simulink library "ddm"  (R2021b)
settings: Solver=VariableStepAuto  StartTime=0.0  StopTime=10.0  RelTol=1e-3
undefined symbols (not defined in the file): ADDM_FrTMTqDev_X_Nm, ADDM_RrTMTqDev_X_Nm, ENUM_ADASACCSTA_ERROR, ENUM_ADASACCSTA_OFF, ENUM_ADASACCSTA_STANDBY, ENUM_ALLOWMOV_ALLOWREADY, ENUM_APS, ENUM_BRKSTA_ERROR, ENUM_BRKSTA_OFF, ENUM_BRKSTA_ON, ENUM_BRKSW_INVALID, ENUM_BRKSW_OFF, ENUM_BRKSW_ON, ENUM_CHGPREACTERRSTA_OBCPRE, ENUM_DCDCFAULTSTA_ANYFAULTLV1, ENUM_DCDCFAULTSTA_ANYFAULTLV2, ENUM_DRIVETRAIN_AWD, ENUM_DRIVETRAIN_FWD, ENUM_DRIVETRAIN_RWD, ENUM_EDUDRTSTA_NORMAL, ENUM_EPBERROR_FAILED, ENUM_EPBSTA_APPLIED, ENUM_EPBSTA_RELEASED, ENUM_ESCAPSSta_APSUNAVAILABLE, ENUM_GEARACTUALPOSN_INVALID, ENUM_GEARACTUALPOSN_P, ENUM_HVBATTREADYPRE_READY, ENUM_HWRESETSTA_HWRESETING, ENUM_MCUWARN_LV0, ENUM_MCUWARN_LV1, ENUM_MCUWARN_LV2, ENUM_MCUWARN_LV3, ENUM_MCUWARN_NOERROR, ENUM_OBCFAULTSTA_ANYFAULT, ENUM_PAS_R2F2, ENUM_PDFAULT_BATTPDFAIL, ENUM_PDFAULT_DCDCDISABLE, ENUM_PDFAULT_MCUDISABLE, ENUM_PDFAULT_MCUDISCHRG, ENUM_POWERSTA_OFF, ENUM_POWERSTA_ON, ENUM_POWERSTA_READY, ENUM_POWERSTA_STANDBY, ENUM_PRESSINDI_LOW, ENUM_PUFAULT_BATTUPFAIL, ENUM_PUFAULT_DCDCENABLEFAIL, ENUM_PUFAULT_PRECHRGCHKFAIL, ENUM_PUFAULT_SAFETYCHKFAIL, ENUM_PWRSTASW_OFF, ENUM_PWRSTASW_OFFA, ENUM_PWRSTASW_OFFCHVCHRG, ENUM_PWRSTASW_OFFCLVCHRG, ENUM_PWRSTASW_ON, ENUM_PWRSTASW_ONHVCHRG, ENUM_PWRSTASW_READY, ENUM_PWRSTASW_STANDBY, ENUM_RAPSErrWarnSta_NORMAL, ENUM_RAPSErrWarnSta_RAPSERRLV1, ENUM_SHIFTCOMMAND_P, ENUM_SHIFTERERRSTA_PBUTTONFAILURE ... (+471)
libraries: hcu_lib x540, simulink x3
(part 16 of 26)

== system ddm/DDM/DDM/VMC_DDM/Enabled Subsystem ==
  task_time_s : Inport
  VPMM_PowerSta_enum : Inport  Port=2
  VDDM_EPS1NoCom_flg : Inport  Port=3
  No_CAN1_BUS_OFF : Inport  Port=4
  DTC_clear_request : Inport  Port=5
  VTQD_GearActualPosn_enum : Inport  Port=6
  VDDM_EPSRCErr_flg : Inport  Port=7
  VDDM_EPSCSErr_flg : Inport  Port=8
  VINP_SASV_flg : Inport  Port=9
  EPS1 Checksum Error : Subsystem
  EPS1 Lost Comm : Subsystem
  "EPS1 Rolling Count Error " : Subsystem
  EPS1 Signal Error : Subsystem
  VDDM_EPS1NoComCFS_flg : Outport
  VDDM_EPS1NoComDTC_raw32 : Outport  Port=2
  VDDM_EPS1RCErrCFS_flg : Outport  Port=3
  VDDM_EPS1RCErrDTC_raw32 : Outport  Port=4
  VDDM_EPS1CSErrCFS_flg : Outport  Port=5
  VDDM_EPS1CSErrDTC_raw32 : Outport  Port=6
  VDDM_EPSSigErrCFS_flg : Outport  Port=7
  VDDM_EPSSigErrDTC_raw32 : Outport  Port=8
  wires:
  [task_time_s] -> EPS1 Lost Comm/1(task_time_s)
  [VPMM_PowerSta_enum] -> EPS1 Lost Comm/2(VPMM_PowerSta_enum)
  [VDDM_EPS1NoCom_flg] -> EPS1 Lost Comm/3(VDDM_EPS1NoCom_flg)
  [No_CAN1_BUS_OFF] -> EPS1 Lost Comm/4(No_CAN1_BUS_OFF)
  [DTC_clear_request] -> EPS1 Lost Comm/5(DTC_clear_request)
  [VTQD_GearActualPosn_enum] -> EPS1 Lost Comm/6(VTQD_GearActualPosn_enum)
  EPS1 Lost Comm/2(VDDM_EPS1NoComDTC_raw32) -> [VDDM_EPS1NoComDTC_raw32]
  EPS1 Lost Comm/1(VDDM_EPS1NoComCFS_flg) -> [VDDM_EPS1NoComCFS_flg]
  task_time_s/1 -> [task_time_s]
  VPMM_PowerSta_enum/1 -> [VPMM_PowerSta_enum]
  VDDM_EPS1NoCom_flg/1 -> [VDDM_EPS1NoCom_flg]
  No_CAN1_BUS_OFF/1 -> [No_CAN1_BUS_OFF]
  DTC_clear_request/1 -> [DTC_clear_request]
  VTQD_GearActualPosn_enum/1 -> [VTQD_GearActualPosn_enum]
  [VDDM_EPS1NoComCFS_flg] -> VDDM_EPS1NoComCFS_flg/1
  [VDDM_EPS1NoComDTC_raw32] -> VDDM_EPS1NoComDTC_raw32/1
  [task_time_s] -> "EPS1 Rolling Count Error "/1(task_time_s)
  [VDDM_EPSRCErr_flg] -> "EPS1 Rolling Count Error "/2(VDDM_EPSRCErr_flg)
  VDDM_EPSRCErr_flg/1 -> [VDDM_EPSRCErr_flg]
  [No_CAN1_BUS_OFF] -> "EPS1 Rolling Count Error "/3(No_CAN1_BUS_OFF)
  [VDDM_EPS1NoComCFS_flg] -> "EPS1 Rolling Count Error "/4(VDDM_EPS1NoComCFS_flg)
  [VPMM_PowerSta_enum] -> "EPS1 Rolling Count Error "/5(VPMM_PowerSta_enum)
  [DTC_clear_request] -> "EPS1 Rolling Count Error "/6(DTC_clear_request)
  [VTQD_GearActualPosn_enum] -> "EPS1 Rolling Count Error "/7(VTQD_GearActualPosn_enum)
  "EPS1 Rolling Count Error "/1(VDDM_EPS1RCErrCFS_flg) -> [VDDM_EPS1RCErrCFS_flg]
  "EPS1 Rolling Count Error "/2(VDDM_EPS1RCErrDTC_raw32) -> [VDDM_EPS1RCErrDTC_raw32]
  [VDDM_EPS1RCErrCFS_flg] -> VDDM_EPS1RCErrCFS_flg/1
  [VDDM_EPS1RCErrDTC_raw32] -> VDDM_EPS1RCErrDTC_raw32/1
  [task_time_s] -> EPS1 Checksum Error/1(task_time_s)
  [VDDM_EPSCSErr_flg] -> EPS1 Checksum Error/2(VDDM_EPSCSErr_flg)
  [No_CAN1_BUS_OFF] -> EPS1 Checksum Error/3(No_CAN1_BUS_OFF)
  [VDDM_EPS1NoComCFS_flg] -> EPS1 Checksum Error/4(VDDM_EPS1NoComCFS_flg)
  [VPMM_PowerSta_enum] -> EPS1 Checksum Error/5(VPMM_PowerSta_enum)
  [DTC_clear_request] -> EPS1 Checksum Error/6(DTC_clear_request)
  [VTQD_GearActualPosn_enum] -> EPS1 Checksum Error/7(VTQD_GearActualPosn_enum)
  VDDM_EPSCSErr_flg/1 -> [VDDM_EPSCSErr_flg]
  EPS1 Checksum Error/1(VDDM_EPS1CSErrCFS_flg) -> [VDDM_EPS1CSErrCFS_flg]
  EPS1 Checksum Error/2(VDDM_EPS1CSErrDTC_raw32) -> [VDDM_EPS1CSErrDTC_raw32]
  [VDDM_EPS1CSErrCFS_flg] -> VDDM_EPS1CSErrCFS_flg/1
  [VDDM_EPS1CSErrDTC_raw32] -> VDDM_EPS1CSErrDTC_raw32/1
  [task_time_s] -> EPS1 Signal Error/1(task_time_s)
  [VINP_SASV_flg] -> EPS1 Signal Error/2(VINP_SASV_flg)
  [No_CAN1_BUS_OFF] -> EPS1 Signal Error/3(No_CAN1_BUS_OFF)
  [VDDM_EPS1NoComCFS_flg] -> EPS1 Signal Error/4(VDDM_EPS1NoComCFS_flg)
  [VPMM_PowerSta_enum] -> EPS1 Signal Error/5(VPMM_PowerSta_enum)
  [DTC_clear_request] -> EPS1 Signal Error/6(DTC_clear_request)
  [VDDM_EPS1RCErrCFS_flg] -> EPS1 Signal Error/7(VDDM_EPS1RCErrCFS_flg)
  [VDDM_EPS1CSErrCFS_flg] -> EPS1 Signal Error/8(VDDM_EPS1CSErrCFS_flg)
  [VTQD_GearActualPosn_enum] -> EPS1 Signal Error/9(VTQD_GearActualPosn_enum)
  EPS1 Signal Error/1(VDDM_EPSSigErrCFS_flg) -> [VDDM_EPSSigErrCFS_flg]
  EPS1 Signal Error/2(VDDM_EPSSigErrDTC_raw32) -> [VDDM_EPSSigErrDTC_raw32]
  [VDDM_EPSSigErrCFS_flg] -> VDDM_EPSSigErrCFS_flg/1
  [VDDM_EPSSigErrDTC_raw32] -> VDDM_EPSSigErrDTC_raw32/1
  VINP_SASV_flg/1 -> [VINP_SASV_flg]

== system ddm/DDM/DDM/VMC_DDM/FCM1 ==
  task_time_s : Inport
  VDDM_FCM1NoCom_flg : Inport  Port=2
  VDDM_FCM1RCErr_flg : Inport  Port=3
  VDDM_FCM1CSErr_flg : Inport  Port=4
  No_CAN6_BUS_OFF : Inport  Port=5
  VPMM_PowerSta_enum : Inport  Port=6
  DTC_clear_request : Inport  Port=7
  "FCM1 Checksum Error " : Subsystem  AncestorBlock=ddm/DDM/DDM/VMC_DDM/FCM2/FCM2 Checksum Error
  FCM1 Lost Com : Subsystem  AncestorBlock=ddm/DDM/DDM/VMC_DDM/FCM2/FCM2 Lost Com
  "FCM1 Rolling Count Error " : Subsystem  AncestorBlock=ddm/DDM/DDM/VMC_DDM/FCM2/FCM2 Rolling Count Error
  VDDM_FCM1NoComCFS_flg : Outport
  VDDM_FCM1RCErrCFS_flg : Outport  Port=2
  VDDM_FCM1CSErrCFS_flg : Outport  Port=3
  VDDM_FCM1NoComDTC_raw32 : Outport  Port=4
  VDDM_FCM1RCErrDTC_raw32 : Outport  Port=5
  VDDM_FCM1CSErrDTC_raw32 : Outport  Port=6
  wires:
  [VDDM_FCM1CSErrDTC_raw32] -> VDDM_FCM1CSErrDTC_raw32/1
  [VDDM_FCM1RCErrDTC_raw32] -> VDDM_FCM1RCErrDTC_raw32/1
  [VDDM_FCM1NoComDTC_raw32] -> VDDM_FCM1NoComDTC_raw32/1
  "FCM1 Checksum Error "/2(VDDM_FCM1CSErrDTC_raw32) -> [VDDM_FCM1CSErrDTC_raw32]
  "FCM1 Rolling Count Error "/2(VDDM_FCM1RCErrDTC_raw32) -> [VDDM_FCM1RCErrDTC_raw32]
  FCM1 Lost Com/2(VDDM_FCM1NoComDTC_raw32) -> [VDDM_FCM1NoComDTC_raw32]
  "FCM1 Checksum Error "/1(VDDM_FCM1CSErrCFS_flg) -> [VDDM_FCM1CSErrCFS_flg]
  [VDDM_FCM1NoComCFS_flg] -> "FCM1 Checksum Error "/4(VDDM_FCM1NoComCFS_flg)
  [VDDM_FCM1CSErr_flg] -> "FCM1 Checksum Error "/2(VDDM_FCM1CSErr_flg)
  [No_CAN6_BUS_OFF] -> "FCM1 Checksum Error "/3(No_CAN6_BUS_OFF)
  [VPMM_PowerSta_enum] -> "FCM1 Checksum Error "/5(VPMM_PowerSta_enum)
  [DTC_clear_request] -> "FCM1 Checksum Error "/6(DTC_clear_request)
  [task_time_s] -> "FCM1 Checksum Error "/1(task_time_s)
  [task_time_s] -> "FCM1 Rolling Count Error "/1(task_time_s)
  task_time_s/1 -> [task_time_s]  "task_time_s"
  [task_time_s] -> FCM1 Lost Com/1(task_time_s)
  VDDM_FCM1CSErr_flg/1 -> [VDDM_FCM1CSErr_flg]
  VDDM_FCM1RCErr_flg/1 -> [VDDM_FCM1RCErr_flg]
  [VDDM_FCM1RCErrCFS_flg] -> VDDM_FCM1RCErrCFS_flg/1
  [VDDM_FCM1CSErrCFS_flg] -> VDDM_FCM1CSErrCFS_flg/1
  [VDDM_FCM1NoComCFS_flg] -> VDDM_FCM1NoComCFS_flg/1
  "FCM1 Rolling Count Error "/1(VDDM_FCM1RCErrCFS_flg) -> [VDDM_FCM1RCErrCFS_flg]
  [DTC_clear_request] -> "FCM1 Rolling Count Error "/6(DTC_clear_request)
  [VPMM_PowerSta_enum] -> "FCM1 Rolling Count Error "/5(VPMM_PowerSta_enum)
  [No_CAN6_BUS_OFF] -> "FCM1 Rolling Count Error "/3(No_CAN6_BUS_OFF)
  [VDDM_FCM1RCErr_flg] -> "FCM1 Rolling Count Error "/2(VDDM_FCM1RCErr_flg)
  [VDDM_FCM1NoComCFS_flg] -> "FCM1 Rolling Count Error "/4(VDDM_FCM1NoComCFS_flg)
  FCM1 Lost Com/1(VDDM_FCM1NoComCFS_flg) -> [VDDM_FCM1NoComCFS_flg]
  [DTC_clear_request] -> FCM1 Lost Com/5(DTC_clear_request)
  [VPMM_PowerSta_enum] -> FCM1 Lost Com/4(VPMM_PowerSta_enum)
  [No_CAN6_BUS_OFF] -> FCM1 Lost Com/3(No_CAN6_BUS_OFF)
  DTC_clear_request/1 -> [DTC_clear_request]
  VPMM_PowerSta_enum/1 -> [VPMM_PowerSta_enum]
  No_CAN6_BUS_OFF/1 -> [No_CAN6_BUS_OFF]
  [VDDM_FCM1NoCom_flg] -> FCM1 Lost Com/2(VDDM_FCM1NoCom_flg)
  VDDM_FCM1NoCom_flg/1 -> [VDDM_FCM1NoCom_flg]

== system ddm/DDM/DDM/VMC_DDM/FCMACC Signal Error ==
  task_time_s : Inport
  VDDM_FCM1NoComCFS_flg : Inport  Port=2
  VDDM_FCM1RCErrCFS_flg : Inport  Port=3
  VDDM_FCM1CSErrCFS_flg : Inport  Port=4
  No_CAN6_BUS_OFF : Inport  Port=5
  VPMM_PowerSta_enum : Inport  Port=6
  VINP_ADASACCSta_enum : Inport  Port=7
  DTC_clear_request : Inport  Port=8
  VTQD_ExternalTqAllow_flg : Inport  Port=9
  VTQD_ExtDoorAllow_flg : Inport  Port=10
  "FCMACC Signal Error " : Subsystem
  VDDM_FCMACCSigErrCFS_flg : Outport
  VDDM_FCMACCSigErrDetDTC_raw32 : Outport  Port=2
  wires:
  VDDM_FCM1CSErrCFS_flg/1 -> [VDDM_FCM1CSErrCFS_flg]
  [VDDM_FCMACCSigErrCFS_flg] -> VDDM_FCMACCSigErrCFS_flg/1
  "FCMACC Signal Error "/1(VDDM_FCMACCSigErrCFS_flg) -> [VDDM_FCMACCSigErrCFS_flg]
  DTC_clear_request/1 -> [DTC_clear_request]
  VPMM_PowerSta_enum/1 -> [VPMM_PowerSta_enum]
  No_CAN6_BUS_OFF/1 -> [No_CAN6_BUS_OFF]
  VDDM_FCM1NoComCFS_flg/1 -> [VDDM_FCM1NoComCFS_flg]
  [No_CAN6_BUS_OFF] -> "FCMACC Signal Error "/5(No_CAN6_BUS_OFF)
  [VPMM_PowerSta_enum] -> "FCMACC Signal Error "/6(VPMM_PowerSta_enum)
  [DTC_clear_request] -> "FCMACC Signal Error "/8(DTC_clear_request)
  task_time_s/1 -> [task_time_s]  "task_time_s"
  [task_time_s] -> "FCMACC Signal Error "/1(task_time_s)
  [VDDM_FCM1NoComCFS_flg] -> "FCMACC Signal Error "/2(VDDM_FCM1NoComCFS_flg)
  [VDDM_FCM1CSErrCFS_flg] -> "FCMACC Signal Error "/4(VDDM_FCM1CSErrCFS_flg)
  VINP_ADASACCSta_enum/1 -> [VINP_ADASACCSta_enum]
  [VINP_ADASACCSta_enum] -> "FCMACC Signal Error "/7(VINP_ADASACCSta_enum)
  "FCMACC Signal Error "/2(VDDM_FCMACCSigErrDetDTC_raw32) -> [VDDM_FCMACCSigErrDetDTC_raw32]
  [VDDM_FCMACCSigErrDetDTC_raw32] -> VDDM_FCMACCSigErrDetDTC_raw32/1
  VTQD_ExternalTqAllow_flg/1 -> [VTQD_ExternalTqAllow_flg]
  VTQD_ExtDoorAllow_flg/1 -> [VTQD_ExtDoorAllow_flg]
  [VTQD_ExternalTqAllow_flg] -> "FCMACC Signal Error "/9(VTQD_ExternalTqAllow_flg)
  [VTQD_ExtDoorAllow_flg] -> "FCMACC Signal Error "/10(VTQD_ExtDoorAllow_flg)
  VDDM_FCM1RCErrCFS_flg/1 -> [VDDM_FCM1RCErrCFS_flg]
  [VDDM_FCM1RCErrCFS_flg] -> "FCMACC Signal Error "/3(VDDM_FCM1RCErrCFS_flg)

== system ddm/DDM/DDM/VMC_DDM/MCU_Fr Signal Error ==
  task_time_s : Inport
  VDDM_MCUF1NoComCFS_flg : Inport  Port=2
  VDDM_MCUF1RCErrCFS_flg : Inport  Port=3
  VDDM_MCUF1CSErrCFS_flg : Inport  Port=4
  No_CAN3_BUS_OFF : Inport  Port=5
  VPMM_PowerSta_enum : Inport  Port=6
  VDDM_MCUWarnF_enum : Inport  Port=7
  DTC_clear_request : Inport  Port=8
  VPMM_DrivetrainSelect_enum : Inport  Port=9
  "MCU_Fr Signal Error " : Subsystem
  VDDM_FrMCUSigErrCFS_flg : Outport
  VDDM_FrMCUSigErrDetDTC_raw32 : Outport  Port=2
  wires:
  [VPMM_DrivetrainSelect_enum] -> "MCU_Fr Signal Error "/9(VPMM_DrivetrainSelect_enum)
  VPMM_DrivetrainSelect_enum/1 -> [VPMM_DrivetrainSelect_enum]
  [VDDM_FrMCUSigErrDetDTC_raw32] -> VDDM_FrMCUSigErrDetDTC_raw32/1
  "MCU_Fr Signal Error "/2(VDDM_FrMCUSigErrDetDTC_raw32) -> [VDDM_FrMCUSigErrDetDTC_raw32]
  [task_time_s] -> "MCU_Fr Signal Error "/1(task_time_s)
  task_time_s/1 -> [task_time_s]  "task_time_s"
  [DTC_clear_request] -> "MCU_Fr Signal Error "/8(DTC_clear_request)
  [VDDM_MCUWarnF_enum] -> "MCU_Fr Signal Error "/7(VDDM_MCUWarnF_enum)
  [VPMM_PowerSta_enum] -> "MCU_Fr Signal Error "/6(VPMM_PowerSta_enum)
  [No_CAN3_BUS_OFF] -> "MCU_Fr Signal Error "/5(No_CAN3_BUS_OFF)
  [VDDM_MCUF1CSErrCFS_flg] -> "MCU_Fr Signal Error "/4(VDDM_MCUF1CSErrCFS_flg)
  [VDDM_MCUF1RCErrCFS_flg] -> "MCU_Fr Signal Error "/3(VDDM_MCUF1RCErrCFS_flg)
  [VDDM_MCUF1NoComCFS_flg] -> "MCU_Fr Signal Error "/2(VDDM_MCUF1NoComCFS_flg)
  VDDM_MCUWarnF_enum/1 -> [VDDM_MCUWarnF_enum]
  VDDM_MCUF1NoComCFS_flg/1 -> [VDDM_MCUF1NoComCFS_flg]
  No_CAN3_BUS_OFF/1 -> [No_CAN3_BUS_OFF]
  VPMM_PowerSta_enum/1 -> [VPMM_PowerSta_enum]
  DTC_clear_request/1 -> [DTC_clear_request]
  "MCU_Fr Signal Error "/1(VDDM_FrMCUSigErrCFS_flg) -> [VDDM_FrMCUSigErrCFS_flg]
  [VDDM_FrMCUSigErrCFS_flg] -> VDDM_FrMCUSigErrCFS_flg/1
  VDDM_MCUF1RCErrCFS_flg/1 -> [VDDM_MCUF1RCErrCFS_flg]
  VDDM_MCUF1CSErrCFS_flg/1 -> [VDDM_MCUF1CSErrCFS_flg]

== system ddm/DDM/DDM/VMC_DDM/MCU_Rr Signal Error ==
  task_time_s : Inport
  VDDM_MCUR1NoComCFS_flg : Inport  Port=2
  VDDM_MCUR1RCErrCFS_flg : Inport  Port=3
  VDDM_MCUR1CSErrCFS_flg : Inport  Port=4
  No_CAN3_BUS_OFF : Inport  Port=5
  VPMM_PowerSta_enum : Inport  Port=6
  VDDM_MCUWarnR_enum : Inport  Port=7
  DTC_clear_request : Inport  Port=8
  VPMM_DrivetrainSelect_enum : Inport  Port=9
  "MCU_Rr Signal Error " : Subsystem
  VDDM_RrMCUSigErrCFS_flg : Outport
  VDDM_RrMCUSigErrDetDTC_raw32 : Outport  Port=2
  wires:
  [VPMM_DrivetrainSelect_enum] -> "MCU_Rr Signal Error "/9(VPMM_DrivetrainSelect_enum)
  VPMM_DrivetrainSelect_enum/1 -> [VPMM_DrivetrainSelect_enum]
  [VDDM_RrMCUSigErrDetDTC_raw32] -> VDDM_RrMCUSigErrDetDTC_raw32/1
  "MCU_Rr Signal Error "/2(VDDM_RrMCUSigErrDetDTC_raw32) -> [VDDM_RrMCUSigErrDetDTC_raw32]
  [task_time_s] -> "MCU_Rr Signal Error "/1(task_time_s)
  task_time_s/1 -> [task_time_s]  "task_time_s"
  [DTC_clear_request] -> "MCU_Rr Signal Error "/8(DTC_clear_request)
  [VDDM_MCUWarnR_enum] -> "MCU_Rr Signal Error "/7(VDDM_MCUWarnR_enum)
  [VPMM_PowerSta_enum] -> "MCU_Rr Signal Error "/6(VPMM_PowerSta_enum)
  [No_CAN3_BUS_OFF] -> "MCU_Rr Signal Error "/5(No_CAN3_BUS_OFF)
  [VDDM_MCUR1CSErrCFS_flg] -> "MCU_Rr Signal Error "/4(VDDM_MCUR1CSErrCFS_flg)
  [VDDM_MCUR1RCErrCFS_flg] -> "MCU_Rr Signal Error "/3(VDDM_MCUR1RCErrCFS_flg)
  [VDDM_MCUR1NoComCFS_flg] -> "MCU_Rr Signal Error "/2(VDDM_MCUR1NoComCFS_flg)
  VDDM_MCUWarnR_enum/1 -> [VDDM_MCUWarnR_enum]
  VDDM_MCUR1NoComCFS_flg/1 -> [VDDM_MCUR1NoComCFS_flg]
  No_CAN3_BUS_OFF/1 -> [No_CAN3_BUS_OFF]
  VPMM_PowerSta_enum/1 -> [VPMM_PowerSta_enum]
  DTC_clear_request/1 -> [DTC_clear_request]
  "MCU_Rr Signal Error "/1(VDDM_RrMCUSigErrCFS_flg) -> [VDDM_RrMCUSigErrCFS_flg]
  [VDDM_RrMCUSigErrCFS_flg] -> VDDM_RrMCUSigErrCFS_flg/1
  VDDM_MCUR1RCErrCFS_flg/1 -> [VDDM_MCUR1RCErrCFS_flg]
  VDDM_MCUR1CSErrCFS_flg/1 -> [VDDM_MCUR1CSErrCFS_flg]

== system ddm/DDM/DDM/VMC_DDM/Shifter Signal Error ==
  task_time_s : Inport
  VDDM_Shifter1NoComCFS_flg : Inport  Port=2
  VDDM_Shifter1RCErrCFS_flg : Inport  Port=3
  VDDM_Shifter1CSErrCFS_flg : Inport  Port=4
  No_CAN3_BUS_OFF : Inport  Port=5
  VPMM_PowerSta_enum : Inport  Port=6
  VINP_ShifterFailsta_enum : Inport  Port=7
  DTC_clear_request : Inport  Port=8
  VTQD_GearActualPosn_enum : Inport  Port=9
  "Shifter Signal Error " : Subsystem
  VDDM_ShifterSigErrCFS_flg : Outport
  VDDM_ShifterSigErrDetDTC_raw32 : Outport  Port=2
  wires:
  [VTQD_GearActualPosn_enum] -> "Shifter Signal Error "/9(VTQD_GearActualPosn_enum)
  VTQD_GearActualPosn_enum/1 -> [VTQD_GearActualPosn_enum]
  [VDDM_ShifterSigErrDetDTC_raw32] -> VDDM_ShifterSigErrDetDTC_raw32/1
  "Shifter Signal Error "/2(VDDM_ShifterSigErrDetDTC_raw32) -> [VDDM_ShifterSigErrDetDTC_raw32]
  [task_time_s] -> "Shifter Signal Error "/1(task_time_s)
  task_time_s/1 -> [task_time_s]  "task_time_s"
  [DTC_clear_request] -> "Shifter Signal Error "/8(DTC_clear_request)
  [VINP_ShifterFailsta_enum] -> "Shifter Signal Error "/7(VINP_ShifterFailsta_enum)
  [VPMM_PowerSta_enum] -> "Shifter Signal Error "/6(VPMM_PowerSta_enum)
  [No_CAN3_BUS_OFF] -> "Shifter Signal Error "/5(No_CAN3_BUS_OFF)
  [VDDM_Shifter1CSErrCFS_flg] -> "Shifter Signal Error "/4(VDDM_Shifter1CSErrCFS_flg)
  [VDDM_Shifter1RCErrCFS_flg] -> "Shifter Signal Error "/3(VDDM_Shifter1RCErrCFS_flg)
  [VDDM_Shifter1NoComCFS_flg] -> "Shifter Signal Error "/2(VDDM_Shifter1NoComCFS_flg)
  VINP_ShifterFailsta_enum/1 -> [VINP_ShifterFailsta_enum]
  VDDM_Shifter1NoComCFS_flg/1 -> [VDDM_Shifter1NoComCFS_flg]
  No_CAN3_BUS_OFF/1 -> [No_CAN3_BUS_OFF]
  VPMM_PowerSta_enum/1 -> [VPMM_PowerSta_enum]
  DTC_clear_request/1 -> [DTC_clear_request]
  "Shifter Signal Error "/1(VDDM_ShifterSigErrCFS_flg) -> [VDDM_ShifterSigErrCFS_flg]
  [VDDM_ShifterSigErrCFS_flg] -> VDDM_ShifterSigErrCFS_flg/1
  VDDM_Shifter1RCErrCFS_flg/1 -> [VDDM_Shifter1RCErrCFS_flg]
  VDDM_Shifter1CSErrCFS_flg/1 -> [VDDM_Shifter1CSErrCFS_flg]

== system ddm/DDM/DDM/VMC_DDM/Zone_Dr_VCU ==
  note: Release Condiction After Decision
  note: Zone_Dr VCU Lost Comm (DrVCUNoCom)
  note: Diagnostics and Fault Handling
  task_time_s : Inport
  VPMM_PowerSta_enum : Inport  Port=2
  No_CAN4_BUS_OFF : Inport  Port=3
  VDDM_DrVCUNoCom_flg : Inport  Port=4
  DTC_clear_request : Inport  Port=5
  Constant : Constant  Value=ENUM_POWERSTA_OFF
  Constant1 : Constant  Value=ENUM_POWERSTA_OFF
  Constant10 : Constant  Value=FALSE
  Constant28 : Constant  Value=KDDM_DrVCUNoComDTC_cnt
  Constant29 : Constant  Value=KDDM_DrVCUNoComPassTO_s
  Constant30 : Constant  Value=KDDM_DrVCUNoComDetTO_s
  Constant4 : Constant  Value=KDDM_VMCDiagnosisOffSW_flg
  Constant49 : Constant  Value=ENUM_POWERSTA_OFF
  Constant5 : Constant  Value=ZERO_INT
  Constant52 : Constant  Value=ENUM_POWERSTA_STANDBY
  Constant55 : Constant  Value=KDDM_DrVCUNoComPassTO_s
  Constant9 : Constant  Value=KDDM_DrVCUNoComDTC_cnt
  DTC_Couter2 : hcu_lib/Basic_Blocks/DTC_Couter
  DTC_Info : hcu_lib/Basic_Blocks/DTC_Info
  Delay : Delay  DelayLength=1
  Equal : RelationalOperator  Operator=~=  OutDataTypeStr=boolean  RndMeth=Simplest
  Equal1 : RelationalOperator  Operator=~=  OutDataTypeStr=boolean  RndMeth=Simplest
  Equal20 : RelationalOperator  OutDataTypeStr=boolean  RndMeth=Simplest
  Equal3 : RelationalOperator  Operator===  OutDataTypeStr=boolean  RndMeth=Simplest
  Equal4 : RelationalOperator  Operator===  OutDataTypeStr=boolean  RndMeth=Simplest
  Logical Operator19 : Logic  Operator=NOT  AllPortsSameDT=off  OutDataTypeStr=boolean
  Logical Operator2 : Logic  AllPortsSameDT=off  OutDataTypeStr=boolean
  Logical Operator3 : Logic  Operator=OR  Inputs=4  AllPortsSameDT=off  OutDataTypeStr=boolean
  Logical Operator4 : Logic  Inputs=3  AllPortsSameDT=off  OutDataTypeStr=boolean
  Logical Operator50 : Logic  Inputs=3  AllPortsSameDT=off  OutDataTypeStr=boolean
  Logical Operator53 : Logic  Operator=NOT  AllPortsSameDT=off  OutDataTypeStr=boolean
  Logical Operator8 : Logic  AllPortsSameDT=off  OutDataTypeStr=boolean
  NOT : Logic  Operator=NOT  AllPortsSameDT=off  OutDataTypeStr=boolean
  Relational Operator : RelationalOperator  Operator=>  OutDataTypeStr=boolean  RndMeth=Simplest
  Switch5 : Switch  Criteria=u2 ~= 0
  Terminator : Terminator
  Test Detection Criteria2 : hcu_lib/Basic_Blocks/Test Detection Criteria
  Timer3 : hcu_lib/Basic_Blocks/Timer
  Unit Delay3 : UnitDelay  SampleTime=-1  HasFrameUpgradeWarning=on
  VDDM_DrVCUNoComCFS_flg : Outport
  VDDM_DrVCUNoComDTC_raw32 : Outport  Port=2
  wires:
  Switch5/1 -> Test Detection Criteria2/1
  Constant10/1 -> Switch5/1
  [VDDM_DrVCUNoComCFSRls_flg] -> Switch5/2
  [VDDM_DrVCUNoComDet_flg] -> DTC_Info/1
  [VDDM_DrVCUNoComPass_flg] -> DTC_Info/2
  [VDDM_DrVCUNoComCFS_flg] -> DTC_Info/3
  [DTC_clear_request] -> DTC_Info/4
  DTC_Info/1 -> [VDDM_DrVCUNoComDTC_raw32]  "VDDM_DrVCUNoComDTC_raw32"
  [VPMM_PowerSta_enum] -> Equal1/1
  Constant1/1 -> Equal1/2
  [VPMM_PowerSta_enum] -> Equal/1
  Constant/1 -> Equal/2
  [VDDM_DrVCUNoCom_flg] -> Logical Operator4/3
  [VDDM_DrVCUNoComCFS_flg] -> Delay/1
  Delay/1 -> NOT/1
  NOT/1 -> Logical Operator2/2
  Constant5/1 -> Relational Operator/2
  DTC_Couter2/1 -> [VDDM_DrVCUNoComCFS_flg]  "VDDM_DrVCUNoComCFS_flg"
  Constant4/1 -> Logical Operator3/4
  [VDDM_DrVCUNoComPass_flg] -> Logical Operator2/1
  Logical Operator2/1 -> Logical Operator3/3
  Equal20/1 -> [VDDM_DrVCUNoComPass_flg]  "VDDM_DrVCUNoComPass_flg"
  Constant52/1 -> Equal4/2
  Unit Delay3/1 -> Equal3/1
  Equal3/1 -> Logical Operator8/1
  Logical Operator4/1 -> Switch5/3
  [No_CAN4_BUS_OFF] -> Logical Operator50/2
  VDDM_DrVCUNoCom_flg/1 -> [VDDM_DrVCUNoCom_flg]
  [No_CAN4_BUS_OFF] -> Logical Operator4/2
  Logical Operator8/1 -> Logical Operator3/1
  Constant9/1 -> DTC_Couter2/3
  No_CAN4_BUS_OFF/1 -> [No_CAN4_BUS_OFF]
  Constant28/1 -> Test Detection Criteria2/3
  task_time_s/1 -> [task_time_s]
  [task_time_s] -> Timer3/3
  Logical Operator50/1 -> Logical Operator19/1, Timer3/1
  [task_time_s] -> Test Detection Criteria2/2
  Relational Operator/1 -> Terminator/1  "VDDM_DrVCUNoComDFS_flg"
  Logical Operator3/1 -> [VDDM_DrVCUNoComCFSRls_flg]  "VDDM_DrVCUNoComCFSRls_flg"
  Logical Operator53/1 -> Logical Operator50/3
  [VPMM_PowerSta_enum] -> Unit Delay3/1
  Equal4/1 -> Logical Operator8/2
  Constant29/1 -> Equal20/2
  DTC_clear_request/1 -> [DTC_clear_request]
  [DTC_clear_request] -> Logical Operator3/2
  Timer3/1 -> Equal20/1
  Logical Operator19/1 -> Timer3/2
  Test Detection Criteria2/1 -> [VDDM_DrVCUNoComDet_flg]  "VDDM_DrVCUNoComDet_flg"
  DTC_Couter2/2 -> Relational Operator/1  "VDDM_DrVCUNoComDTC_cnt"
  Constant49/1 -> Equal3/2
  VPMM_PowerSta_enum/1 -> [VPMM_PowerSta_enum]
  Constant55/1 -> Timer3/4
  [VDDM_DrVCUNoComDet_flg] -> DTC_Couter2/1
  Constant30/1 -> Test Detection Criteria2/4
  [VPMM_PowerSta_enum] -> Equal4/1
  [VDDM_DrVCUNoComCFSRls_flg] -> DTC_Couter2/2
  Equal/1 -> Logical Operator4/1
  Equal1/1 -> Logical Operator50/1
  [VDDM_DrVCUNoComDTC_raw32] -> VDDM_DrVCUNoComDTC_raw32/1
  [VDDM_DrVCUNoComCFS_flg] -> VDDM_DrVCUNoComCFS_flg/1
  [VDDM_DrVCUNoCom_flg] -> Logical Operator53/1

== system ddm/DDM/DDM/VMC_DDM/Zone_Fr_VCU ==
  note: Diagnostics and Fault Handling
  note: Zone_Fr VCU Lost Comm (FrVCUNoCom)
  note: Release Condiction After Decision
  task_time_s : Inport
  VPMM_PowerSta_enum : Inport  Port=2
  No_CAN4_BUS_OFF : Inport  Port=3
  VDDM_FrVCUNoCom_flg : Inport  Port=4
  DTC_clear_request : Inport  Port=5
  Constant : Constant  Value=ENUM_POWERSTA_OFF
  Constant1 : Constant  Value=ENUM_POWERSTA_OFF
  Constant10 : Constant  Value=FALSE
  Constant28 : Constant  Value=KDDM_FrVCUNoComDTC_cnt
  Constant29 : Constant  Value=KDDM_FrVCUNoComPassTO_s
  Constant30 : Constant  Value=KDDM_FrVCUNoComDetTO_s
  Constant4 : Constant  Value=KDDM_VMCDiagnosisOffSW_flg
  Constant49 : Constant  Value=ENUM_POWERSTA_OFF
  Constant5 : Constant  Value=ZERO_INT
  Constant52 : Constant  Value=ENUM_POWERSTA_STANDBY
  Constant55 : Constant  Value=KDDM_FrVCUNoComPassTO_s
  Constant9 : Constant  Value=KDDM_FrVCUNoComDTC_cnt
  DTC_Couter2 : hcu_lib/Basic_Blocks/DTC_Couter
  DTC_Info : hcu_lib/Basic_Blocks/DTC_Info
  Delay : Delay  DelayLength=1
  Equal : RelationalOperator  Operator=~=  OutDataTypeStr=boolean  RndMeth=Simplest
  Equal1 : RelationalOperator  Operator=~=  OutDataTypeStr=boolean  RndMeth=Simplest
  Equal20 : RelationalOperator  OutDataTypeStr=boolean  RndMeth=Simplest
  Equal3 : RelationalOperator  Operator===  OutDataTypeStr=boolean  RndMeth=Simplest
  Equal4 : RelationalOperator  Operator===  OutDataTypeStr=boolean  RndMeth=Simplest
  Logical Operator19 : Logic  Operator=NOT  AllPortsSameDT=off  OutDataTypeStr=boolean
  Logical Operator2 : Logic  AllPortsSameDT=off  OutDataTypeStr=boolean
  Logical Operator3 : Logic  Operator=OR  Inputs=4  AllPortsSameDT=off  OutDataTypeStr=boolean
  Logical Operator4 : Logic  Inputs=3  AllPortsSameDT=off  OutDataTypeStr=boolean
  Logical Operator50 : Logic  Inputs=3  AllPortsSameDT=off  OutDataTypeStr=boolean
  Logical Operator53 : Logic  Operator=NOT  AllPortsSameDT=off  OutDataTypeStr=boolean
  Logical Operator8 : Logic  AllPortsSameDT=off  OutDataTypeStr=boolean
  NOT : Logic  Operator=NOT  AllPortsSameDT=off  OutDataTypeStr=boolean
  Relational Operator : RelationalOperator  Operator=>  OutDataTypeStr=boolean  RndMeth=Simplest
  Switch5 : Switch  Criteria=u2 ~= 0
  Terminator : Terminator
  Test Detection Criteria2 : hcu_lib/Basic_Blocks/Test Detection Criteria
  Timer3 : hcu_lib/Basic_Blocks/Timer
  Unit Delay3 : UnitDelay  SampleTime=-1  HasFrameUpgradeWarning=on
  VDDM_FrVCUNoComCFS_flg : Outport
  VDDM_FrVCUNoComDTC_raw32 : Outport  Port=2
  wires:
  [DTC_clear_request] -> DTC_Info/4
  [VDDM_FrVCUNoComDet_flg] -> DTC_Info/1
  [VDDM_FrVCUNoComPass_flg] -> DTC_Info/2
  [VDDM_FrVCUNoComCFS_flg] -> DTC_Info/3
  DTC_Info/1 -> [VDDM_FrVCUNoComDTC_raw32]  "VDDM_FrVCUNoComDTC_raw32"
  Switch5/1 -> Test Detection Criteria2/1
  Constant10/1 -> Switch5/1
  [VDDM_FrVCUNoComCFSRls_flg] -> Switch5/2
  Constant1/1 -> Equal1/2
  [VPMM_PowerSta_enum] -> Equal1/1
  Constant/1 -> Equal/2
  [VPMM_PowerSta_enum] -> Equal/1
  [VDDM_FrVCUNoCom_flg] -> Logical Operator53/1
  [VDDM_FrVCUNoComCFS_flg] -> VDDM_FrVCUNoComCFS_flg/1
  [VDDM_FrVCUNoComDTC_raw32] -> VDDM_FrVCUNoComDTC_raw32/1
  Equal1/1 -> Logical Operator50/1
  Equal/1 -> Logical Operator4/1
  [VDDM_FrVCUNoComCFSRls_flg] -> DTC_Couter2/2
  [VPMM_PowerSta_enum] -> Equal4/1
  Constant30/1 -> Test Detection Criteria2/4
  [VDDM_FrVCUNoComDet_flg] -> DTC_Couter2/1
  Constant55/1 -> Timer3/4
  VPMM_PowerSta_enum/1 -> [VPMM_PowerSta_enum]
  Constant49/1 -> Equal3/2
  DTC_Couter2/2 -> Relational Operator/1  "VDDM_FrVCUNoComDTC_cnt"
  Test Detection Criteria2/1 -> [VDDM_FrVCUNoComDet_flg]  "VDDM_FrVCUNoComDet_flg"
  Logical Operator19/1 -> Timer3/2
  Timer3/1 -> Equal20/1
  [DTC_clear_request] -> Logical Operator3/2
  DTC_clear_request/1 -> [DTC_clear_request]
  Constant29/1 -> Equal20/2
  Equal4/1 -> Logical Operator8/2
  [VPMM_PowerSta_enum] -> Unit Delay3/1
  Logical Operator53/1 -> Logical Operator50/3
  Logical Operator3/1 -> [VDDM_FrVCUNoComCFSRls_flg]  "VDDM_FrVCUNoComCFSRls_flg"
  Relational Operator/1 -> Terminator/1  "VDDM_FrVCUNoComDFS_flg"
  [task_time_s] -> Test Detection Criteria2/2
  Logical Operator50/1 -> Timer3/1, Logical Operator19/1
  [task_time_s] -> Timer3/3
  task_time_s/1 -> [task_time_s]
  Constant28/1 -> Test Detection Criteria2/3
  No_CAN4_BUS_OFF/1 -> [No_CAN4_BUS_OFF]
  Constant9/1 -> DTC_Couter2/3
  Logical Operator8/1 -> Logical Operator3/1
  [No_CAN4_BUS_OFF] -> Logical Operator4/2
  VDDM_FrVCUNoCom_flg/1 -> [VDDM_FrVCUNoCom_flg]
  [No_CAN4_BUS_OFF] -> Logical Operator50/2
  Logical Operator4/1 -> Switch5/3
  Equal3/1 -> Logical Operator8/1
  Unit Delay3/1 -> Equal3/1
  Constant52/1 -> Equal4/2
  Equal20/1 -> [VDDM_FrVCUNoComPass_flg]  "VDDM_FrVCUNoComPass_flg"
  Logical Operator2/1 -> Logical Operator3/3
  [VDDM_FrVCUNoComPass_flg] -> Logical Operator2/1
  Constant4/1 -> Logical Operator3/4
  DTC_Couter2/1 -> [VDDM_FrVCUNoComCFS_flg]  "VDDM_FrVCUNoComCFS_flg"
  Constant5/1 -> Relational Operator/2
  NOT/1 -> Logical Operator2/2
  Delay/1 -> NOT/1
  [VDDM_FrVCUNoComCFS_flg] -> Delay/1
  [VDDM_FrVCUNoCom_flg] -> Logical Operator4/3

== system ddm/DDM/DDM/VMC_DDM/Zone_dr Error ==
  task_time_s : Inport
  VDDM_DrVCUNoComCFS_flg : Inport  Port=2
  No_CAN4_BUS_OFF : Inport  Port=3
  VPMM_PowerSta_enum : Inport  Port=4
  VINP_ZoneDrMalfunLevel_enum : Inport  Port=5
  DTC_clear_request : Inport  Port=6
  "Zone_dr Error " : Subsystem
  VDDM_ZoneDrSigErrCFS_flg : Outport
  VDDM_ZoneDrSigErrDetDTC_raw32 : Outport  Port=2
  wires:
  [VDDM_ZoneDrSigErrDetDTC_raw32] -> VDDM_ZoneDrSigErrDetDTC_raw32/1
  "Zone_dr Error "/2(VDDM_ZoneDrSigErrDetDTC_raw32) -> [VDDM_ZoneDrSigErrDetDTC_raw32]
  [task_time_s] -> "Zone_dr Error "/1(task_time_s)
  task_time_s/1 -> [task_time_s]  "task_time_s"
  [DTC_clear_request] -> "Zone_dr Error "/6(DTC_clear_request)
  [VINP_ZoneDrMalfunLevel_enum] -> "Zone_dr Error "/5(VINP_ZoneDrMalfunLevel_enum)
  [VPMM_PowerSta_enum] -> "Zone_dr Error "/4(VPMM_PowerSta_enum)
  [No_CAN4_BUS_OFF] -> "Zone_dr Error "/3(No_CAN4_BUS_OFF)
  [VDDM_DrVCUNoComCFS_flg] -> "Zone_dr Error "/2(VDDM_DrVCUNoComCFS_flg)
  VINP_ZoneDrMalfunLevel_enum/1 -> [VINP_ZoneDrMalfunLevel_enum]
  VDDM_DrVCUNoComCFS_flg/1 -> [VDDM_DrVCUNoComCFS_flg]
  No_CAN4_BUS_OFF/1 -> [No_CAN4_BUS_OFF]
  VPMM_PowerSta_enum/1 -> [VPMM_PowerSta_enum]
  DTC_clear_request/1 -> [DTC_clear_request]
  "Zone_dr Error "/1(VDDM_ZoneDrSigErrCFS_flg) -> [VDDM_ZoneDrSigErrCFS_flg]
  [VDDM_ZoneDrSigErrCFS_flg] -> VDDM_ZoneDrSigErrCFS_flg/1

== system ddm/DDM/DDM/VMC_DDM/Zone_fr Error ==
  task_time_s : Inport
  VDDM_FrVCUNoComCFS_flg : Inport  Port=2
  No_CAN4_BUS_OFF : Inport  Port=3
  VPMM_PowerSta_enum : Inport  Port=4
  ZoneFrMalfunLevel_enum : Inport  Port=5
  DTC_clear_request : Inport  Port=6
  "Zone_fr Error " : Subsystem
  VDDM_ZoneFrSigErrCFS_flg : Outport
  VDDM_ZoneFrSigErrDetDTC_raw32 : Outport  Port=2
  wires:
  [VDDM_ZoneFrSigErrCFS_flg] -> VDDM_ZoneFrSigErrCFS_flg/1
  "Zone_fr Error "/1(VDDM_ZoneFrSigErrCFS_flg) -> [VDDM_ZoneFrSigErrCFS_flg]
  DTC_clear_request/1 -> [DTC_clear_request]
  VPMM_PowerSta_enum/1 -> [VPMM_PowerSta_enum]
  No_CAN4_BUS_OFF/1 -> [No_CAN4_BUS_OFF]
  VDDM_FrVCUNoComCFS_flg/1 -> [VDDM_FrVCUNoComCFS_flg]
  ZoneFrMalfunLevel_enum/1 -> [ZoneFrMalfunLevel_enum]
  [VDDM_FrVCUNoComCFS_flg] -> "Zone_fr Error "/2(VDDM_FrVCUNoComCFS_flg)
  [No_CAN4_BUS_OFF] -> "Zone_fr Error "/3(No_CAN4_BUS_OFF)
  [VPMM_PowerSta_enum] -> "Zone_fr Error "/4(VPMM_PowerSta_enum)
  [ZoneFrMalfunLevel_enum] -> "Zone_fr Error "/5(ZoneFrMalfunLevel_enum)
  [DTC_clear_request] -> "Zone_fr Error "/6(DTC_clear_request)
  task_time_s/1 -> [task_time_s]  "task_time_s"
  [task_time_s] -> "Zone_fr Error "/1(task_time_s)
  "Zone_fr Error "/2(VDDM_ZoneFrSigErrDetDTC_raw32) -> [VDDM_ZoneFrSigErrDetDTC_raw32]
  [VDDM_ZoneFrSigErrDetDTC_raw32] -> VDDM_ZoneFrSigErrDetDTC_raw32/1

== system ddm/DDM/DDM/PMM/Brake switch signal abnormal1/Brake switch signal abnormal ==
  note: Test Pass Criteria
  note: Diagnostics and Fault Handling
  note: Test Detection Criteria
  note: Release Condition After Decision
  task_time_s : Inport
  VPMM_PowerSta_enum : Inport  Port=2
  BrkSWErr : Inport  Port=3
  DTC_clear_request : Inport  Port=4
  VINP_BrkPedalPos_pct : Inport  Port=5
  VDDM_ESC5Err_flg : Inport  Port=6
  Constant1 : Constant  Value=TRUE
  Constant10 : Constant  Value=ENUM_POWERSTA_STANDBY
  Constant12 : Constant  Value=FALSE
  Constant14 : Constant  Value=KDDM_BrkSWErrDetTO_s
  Constant17 : Constant  Value=KDDM_BrkSWErrDTC_cnt
  Constant18 : Constant  Value=KDDM_BrkSWErrDTC_cnt
  Constant2 : Constant  Value=KDDM_UpDetWinBrkPos_pct
  Constant3 : Constant  Value=KDDM_DwnDetWinBrkPos_pct
  Constant30 : Constant  Value=KDDM_BrkSWDiagnosisOffSW_flg
  Constant31 : Constant  Value=ENUM_POWERSTA_OFF
  Constant33 : Constant  Value=KDDM_BrkSWErrPassTO_s
  Constant34 : Constant  Value=KDDM_BrkSWErrPassTO_s
  Constant4 : Constant  Value=KDDM_UpDetWinBrkPos_pct
  Constant5 : Constant  Value=KDDM_DwnDetWinBrkPos_pct
  Constant6 : Constant  Value=FALSE
  Constant7 : Constant  Value=ENUM_PWRSTASW_OFF
  Constant8 : Constant  Value=ENUM_PWRSTASW_OFF
  Constant9 : Constant  Value=ZERO_INT
  DTC_Couter1 : hcu_lib/Basic_Blocks/DTC_Couter
  DTC_Info : hcu_lib/Basic_Blocks/DTC_Info
  Equal1 : RelationalOperator  OutDataTypeStr=boolean  RndMeth=Simplest
  Equal10 : RelationalOperator  Operator===  OutDataTypeStr=boolean  RndMeth=Simplest
  Equal2 : RelationalOperator  OutDataTypeStr=boolean  RndMeth=Simplest
  Equal3 : RelationalOperator  Operator=<=  OutDataTypeStr=boolean  RndMeth=Simplest
  Equal4 : RelationalOperator  Operator=<=  OutDataTypeStr=boolean  RndMeth=Simplest
  Equal8 : RelationalOperator  OutDataTypeStr=boolean  RndMeth=Simplest
  Equal9 : RelationalOperator  Operator===  OutDataTypeStr=boolean  RndMeth=Simplest
  Logical Operator : Logic  Operator=NOT  AllPortsSameDT=off  OutDataTypeStr=boolean
  Logical Operator1 : Logic  Inputs=3  AllPortsSameDT=off  OutDataTypeStr=boolean
  Logical Operator16 : Logic  Operator=OR  Inputs=4  AllPortsSameDT=off  OutDataTypeStr=boolean
  Logical Operator17 : Logic  AllPortsSameDT=off  OutDataTypeStr=boolean
  Logical Operator2 : Logic  Operator=OR  AllPortsSameDT=off  OutDataTypeStr=boolean
  Logical Operator21 : Logic  Operator=NOT  AllPortsSameDT=off  OutDataTypeStr=boolean
  Logical Operator3 : Logic  Inputs=3  AllPortsSameDT=off  OutDataTypeStr=boolean
  Logical Operator4 : Logic  Operator=OR  AllPortsSameDT=off  OutDataTypeStr=boolean
  Logical Operator5 : Logic  Operator=NOT  AllPortsSameDT=off  OutDataTypeStr=boolean
  NotEqual : RelationalOperator  Operator=~=  OutDataTypeStr=boolean  RndMeth=Simplest
  NotEqual1 : RelationalOperator  Operator=~=  OutDataTypeStr=boolean  RndMeth=Simplest
  Relational Operator1 : RelationalOperator  Operator=>  OutDataTypeStr=boolean  RndMeth=Simplest
  Switch1 : Switch  Criteria=u2 ~= 0
  Switch2 : Switch  Criteria=u2 ~= 0
  Switch9 : Switch  Criteria=u2 ~= 0
  Terminator : Terminator
  Test Detection Criteria1 : hcu_lib/Basic_Blocks/Test Detection Criteria
  Timer2 : hcu_lib/Basic_Blocks/Timer
  Unit Delay1 : UnitDelay  SampleTime=-1  HasFrameUpgradeWarning=on
  VDDM_BrkSWErrDTC_raw32 : Outport
  VDDM_BrkSWErrCFS_flg : Outport  Port=2
  wires:
  VINP_BrkPedalPos_pct/1 -> [VINP_BrkPedalPos_pct]
  [DTC_clear_request] -> DTC_Info/4
  [VDDM_BrkSWErrDet_flg] -> DTC_Info/1
  BrkSWErr/1 -> [BrkSWErr]
  [VDDM_BrkSWErrCFS_flg] -> DTC_Info/3
  [VDDM_BrkSWErrPass_flg] -> DTC_Info/2
  DTC_Info/1 -> VDDM_BrkSWErrDTC_raw32/1  "VDDM_BrkSWErrDTC_raw32"
  DTC_clear_request/1 -> [DTC_clear_request]
  task_time_s/1 -> [task_time_s]
  VPMM_PowerSta_enum/1 -> [VPMM_PowerSta_enum]
  [VDDM_BrkSWErrPass_flg] -> Logical Operator16/3
  Constant14/1 -> Test Detection Criteria1/4
  Equal8/1 -> [VDDM_BrkSWErrPass_flg]  "VDDM_BrkSWErrPass_flg"
  Constant18/1 -> DTC_Couter1/3
  Constant17/1 -> Test Detection Criteria1/3
  Constant33/1 -> Timer2/4
  Test Detection Criteria1/1 -> [VDDM_BrkSWErrDet_flg]  "VDDM_BrkSWErrDet_flg"
  Constant10/1 -> Equal10/2
  Timer2/1 -> Equal8/1
  Constant6/1 -> Switch9/1
  [VPMM_PowerSta_enum] -> Equal10/1
  [BrkSWErr] -> Switch1/1
  DTC_Couter1/2 -> Relational Operator1/1  "VDDM_BrkSWErrDTC_cnt"
  [DTC_clear_request] -> Logical Operator16/2
  Constant31/1 -> Equal9/2
  Equal10/1 -> Logical Operator17/2
  Constant12/1 -> Switch1/3
  Logical Operator17/1 -> Logical Operator16/1
  Logical Operator21/1 -> Timer2/1
  Switch1/1 -> Switch9/3
  [task_time_s] -> Timer2/3
  [task_time_s] -> Test Detection Criteria1/2
  Switch9/1 -> Test Detection Criteria1/1
  Constant30/1 -> Logical Operator16/4
  Switch2/1 -> Timer2/2, Logical Operator21/1
  Equal9/1 -> Logical Operator17/1
  [VPMM_PowerSta_enum] -> Unit Delay1/1
  Constant9/1 -> Relational Operator1/2
  Relational Operator1/1 -> Terminator/1  "VDDM_BrkSWErrDFS_flg"
  Unit Delay1/1 -> Equal9/1
  [VDDM_BrkSWErrCFSRls_flg] -> Switch9/2
  Constant34/1 -> Equal8/2
  DTC_Couter1/1 -> [VDDM_BrkSWErrCFS_flg]  "VDDM_BrkSWErrCFS_flg"
  [VDDM_BrkSWErrDet_flg] -> DTC_Couter1/1
  [VDDM_BrkSWErrCFSRls_flg] -> DTC_Couter1/2
  Logical Operator16/1 -> [VDDM_BrkSWErrCFSRls_flg]  "VDDM_BrkSWErrCFSRls_flg"
  [VDDM_BrkSWErrCFS_flg] -> VDDM_BrkSWErrCFS_flg/1
  Equal2/1 -> Logical Operator2/1
  Logical Operator1/1 -> Switch1/2
  [VPMM_PowerSta_enum] -> NotEqual/1
  Constant3/1 -> Equal3/2
  Constant2/1 -> Equal2/2
  Constant7/1 -> NotEqual/2
  Logical Operator2/1 -> Logical Operator1/2
  [VINP_BrkPedalPos_pct] -> Equal3/1
  [VINP_BrkPedalPos_pct] -> Equal2/1
  NotEqual/1 -> Logical Operator1/1
  Equal3/1 -> Logical Operator2/2
  VDDM_ESC5Err_flg/1 -> [VDDM_ESC5Err_flg]
  [VDDM_ESC5Err_flg] -> Logical Operator/1
  Constant5/1 -> Equal4/2
  Equal4/1 -> Logical Operator4/2
  [VPMM_PowerSta_enum] -> NotEqual1/1
  Logical Operator4/1 -> Logical Operator3/2
  Constant8/1 -> NotEqual1/2
  [VINP_BrkPedalPos_pct] -> Equal4/1
  NotEqual1/1 -> Logical Operator3/1
  Constant4/1 -> Equal1/2
  Logical Operator3/1 -> Switch2/2
  Constant1/1 -> Switch2/3
  [VINP_BrkPedalPos_pct] -> Equal1/1
  Equal1/1 -> Logical Operator4/1
  [BrkSWErr] -> Switch2/1
  Logical Operator/1 -> Logical Operator1/3
  [VDDM_ESC5Err_flg] -> Logical Operator5/1
  Logical Operator5/1 -> Logical Operator3/3

== system ddm/DDM/DDM/PMM/Brake switch signal abnormal1/Brake switch signal abnormal and no backup signal ==
  note: Diagnostics and Fault Handling
  note: Release Condition After Decision
  note: Test Pass Criteria
  note: Test Detection Criteria
  task_time_s : Inport
  VPMM_PowerSta_enum : Inport  Port=2
  BrkSWNoBac : Inport  Port=3
  DTC_clear_request : Inport  Port=4
  VINP_BrkPedalPos_pct : Inport  Port=5
  VDDM_ESC5Err_flg : Inport  Port=6
  Constant1 : Constant  Value=ENUM_PWRSTASW_OFF
  Constant10 : Constant  Value=ENUM_POWERSTA_STANDBY
  Constant12 : Constant  Value=FALSE
  Constant14 : Constant  Value=KDDM_BrkSWNoBacDetTO_s
  Constant17 : Constant  Value=KDDM_BrkSWNoBacDTC_cnt
  Constant18 : Constant  Value=KDDM_BrkSWNoBacPassTO_s
  Constant2 : Constant  Value=KDDM_UpDetWinBrkPos_pct
  Constant21 : Constant  Value=ZERO_INT
  Constant22 : Constant  Value=KDDM_BrkSWNoBacPassTO_s
  Constant3 : Constant  Value=KDDM_DwnDetWinBrkPos_pct
  Constant30 : Constant  Value=KDDM_BrkSWDiagnosisOffSW_flg
  Constant31 : Constant  Value=ENUM_POWERSTA_OFF
  Constant33 : Constant  Value=KDDM_BrkSWNoBacDTC_cnt
  Constant4 : Constant  Value=TRUE
  Constant5 : Constant  Value=ENUM_PWRSTASW_OFF
  Constant6 : Constant  Value=KDDM_UpDetWinBrkPos_pct
  Constant7 : Constant  Value=FALSE
  Constant8 : Constant  Value=KDDM_DwnDetWinBrkPos_pct
  DTC_Couter1 : hcu_lib/Basic_Blocks/DTC_Couter
  DTC_Info : hcu_lib/Basic_Blocks/DTC_Info
  Delay1 : Delay  DelayLength=1
  Equal1 : RelationalOperator  OutDataTypeStr=boolean  RndMeth=Simplest
  Equal10 : RelationalOperator  Operator===  OutDataTypeStr=boolean  RndMeth=Simplest
  Equal14 : RelationalOperator  OutDataTypeStr=boolean  RndMeth=Simplest
  Equal15 : RelationalOperator  Operator===  OutDataTypeStr=boolean  RndMeth=Simplest
  Equal2 : RelationalOperator  OutDataTypeStr=boolean  RndMeth=Simplest
  Equal3 : RelationalOperator  Operator=<=  OutDataTypeStr=boolean  RndMeth=Simplest
  Equal4 : RelationalOperator  Operator=<=  OutDataTypeStr=boolean  RndMeth=Simplest
  Logical Operator : Logic  Operator=NOT  AllPortsSameDT=off  OutDataTypeStr=boolean
  Logical Operator1 : Logic  Inputs=3  AllPortsSameDT=off  OutDataTypeStr=boolean
  Logical Operator11 : Logic  AllPortsSameDT=off  OutDataTypeStr=boolean
  Logical Operator16 : Logic  Operator=OR  Inputs=4  AllPortsSameDT=off  OutDataTypeStr=boolean
  Logical Operator17 : Logic  AllPortsSameDT=off  OutDataTypeStr=boolean
  Logical Operator2 : Logic  Operator=OR  AllPortsSameDT=off  OutDataTypeStr=boolean
  Logical Operator21 : Logic  Operator=NOT  AllPortsSameDT=off  OutDataTypeStr=boolean
  Logical Operator3 : Logic  Inputs=3  AllPortsSameDT=off  OutDataTypeStr=boolean
  Logical Operator4 : Logic  Operator=OR  AllPortsSameDT=off  OutDataTypeStr=boolean
  Logical Operator5 : Logic  Operator=NOT  AllPortsSameDT=off  OutDataTypeStr=boolean
  NOT1 : Logic  Operator=NOT  AllPortsSameDT=off  OutDataTypeStr=boolean
  NotEqual : RelationalOperator  Operator=~=  OutDataTypeStr=boolean  RndMeth=Simplest
  NotEqual1 : RelationalOperator  Operator=~=  OutDataTypeStr=boolean  RndMeth=Simplest
  Relational Operator1 : RelationalOperator  Operator=>  OutDataTypeStr=boolean  RndMeth=Simplest
  Switch1 : Switch  Criteria=u2 ~= 0
  Switch2 : Switch  Criteria=u2 ~= 0
  Switch9 : Switch  Criteria=u2 ~= 0
  Terminator : Terminator
  Test Detection Criteria1 : hcu_lib/Basic_Blocks/Test Detection Criteria
  Timer2 : hcu_lib/Basic_Blocks/Timer
  Unit Delay1 : UnitDelay  SampleTime=-1  HasFrameUpgradeWarning=on
  VDDM_BrkSWNoBacDTC_raw32 : Outport
  VDDM_BrkSWNoBacCFS_flg : Outport  Port=2
  wires:
  VINP_BrkPedalPos_pct/1 -> [VINP_BrkPedalPos_pct]
  Constant4/1 -> Switch2/3
  Logical Operator1/1 -> Switch1/2
  Constant12/1 -> Switch1/3
  [DTC_clear_request] -> DTC_Info/4
  [VDDM_BrkSWNoBacDet_flg] -> DTC_Info/1
  BrkSWNoBac/1 -> [BrkSWNoBac]
  [VDDM_BrkSWNoBacCFS_flg] -> DTC_Info/3
  [VDDM_BrkSWNoBacPass_flg] -> DTC_Info/2
  DTC_Info/1 -> VDDM_BrkSWNoBacDTC_raw32/1  "VDDM_BrkSWNoBacDTC_raw32"
  DTC_clear_request/1 -> [DTC_clear_request]
  VPMM_PowerSta_enum/1 -> [VPMM_PowerSta_enum]
  task_time_s/1 -> [task_time_s]
  Constant33/1 -> DTC_Couter1/3
  [BrkSWNoBac] -> Switch1/1
  [VDDM_BrkSWNoBacCFSRls_flg] -> DTC_Couter1/2
  [VDDM_BrkSWNoBacDet_flg] -> DTC_Couter1/1
  Logical Operator16/1 -> [VDDM_BrkSWNoBacCFSRls_flg]  "VDDM_BrkSWNoBacCFSRls_flg"
  Equal15/1 -> Logical Operator17/1
  Switch2/1 -> Logical Operator21/1, Timer2/2
  Switch9/1 -> Test Detection Criteria1/1
  Switch1/1 -> Switch9/3
  [task_time_s] -> Test Detection Criteria1/2
  [task_time_s] -> Timer2/3
  Constant31/1 -> Equal15/2
  Equal10/1 -> Logical Operator17/2
  [VPMM_PowerSta_enum] -> Unit Delay1/1
  [VPMM_PowerSta_enum] -> Equal10/1
  Constant7/1 -> Switch9/1
  Timer2/1 -> Equal14/1
  Logical Operator21/1 -> Timer2/1
  Constant22/1 -> Equal14/2
  DTC_Couter1/1 -> [VDDM_BrkSWNoBacCFS_flg]  "VDDM_BrkSWNoBacCFS_flg"
  Equal14/1 -> [VDDM_BrkSWNoBacPass_flg]  "VDDM_BrkSWNoBacPass_flg"
  Relational Operator1/1 -> Terminator/1  "VDDM_BrkSWNoBacDFS_flg"
  [VDDM_BrkSWNoBacCFSRls_flg] -> Switch9/2
  Logical Operator17/1 -> Logical Operator16/1
  Constant21/1 -> Relational Operator1/2
  Test Detection Criteria1/1 -> [VDDM_BrkSWNoBacDet_flg]  "VDDM_BrkSWNoBacDet_flg"
  Constant17/1 -> Test Detection Criteria1/3
  [BrkSWNoBac] -> Switch2/1
  [DTC_clear_request] -> Logical Operator16/2
  DTC_Couter1/2 -> Relational Operator1/1  "VDDM_BrkSWNoBacDTC_cnt"
  Constant14/1 -> Test Detection Criteria1/4
  Constant30/1 -> Logical Operator16/4
  Unit Delay1/1 -> Equal15/1
  Constant10/1 -> Equal10/2
  Constant18/1 -> Timer2/4
  [VDDM_BrkSWNoBacPass_flg] -> Logical Operator11/1
  Delay1/1 -> NOT1/1
  NOT1/1 -> Logical Operator11/2
  [VDDM_BrkSWNoBacCFS_flg] -> Delay1/1
  Logical Operator11/1 -> Logical Operator16/3
  [VDDM_BrkSWNoBacCFS_flg] -> VDDM_BrkSWNoBacCFS_flg/1
  Equal3/1 -> Logical Operator2/2
  [VINP_BrkPedalPos_pct] -> Equal2/1
  [VINP_BrkPedalPos_pct] -> Equal3/1
  [VPMM_PowerSta_enum] -> NotEqual/1
  Equal2/1 -> Logical Operator2/1
  NotEqual/1 -> Logical Operator1/1
  Logical Operator2/1 -> Logical Operator1/2
  Constant1/1 -> NotEqual/2
  Constant3/1 -> Equal3/2
  Constant2/1 -> Equal2/2
  Equal4/1 -> Logical Operator4/2
  [VINP_BrkPedalPos_pct] -> Equal1/1
  [VINP_BrkPedalPos_pct] -> Equal4/1
  [VPMM_PowerSta_enum] -> NotEqual1/1
  Equal1/1 -> Logical Operator4/1
  NotEqual1/1 -> Logical Operator3/1
  Logical Operator4/1 -> Logical Operator3/2
  Constant5/1 -> NotEqual1/2
  Logical Operator3/1 -> Switch2/2
  Constant8/1 -> Equal4/2
  Constant6/1 -> Equal1/2
  VDDM_ESC5Err_flg/1 -> [VDDM_ESC5Err_flg]
  [VDDM_ESC5Err_flg] -> Logical Operator/1
  Logical Operator/1 -> Logical Operator1/3
  [VDDM_ESC5Err_flg] -> Logical Operator5/1
  Logical Operator5/1 -> Logical Operator3/3
